simulink model "watertank_inport_NN_cex"  (R2019a)
settings: Solver=FixedStepAuto  StartTime=0.0  StopTime=options.T_train  FixedStep=0.01  RelTol=1e-3
model workspace (MAT data in the model file):
  A = 20
  a = 2
  b = 5
undefined symbols (not defined in the file): options
libraries: neural x132, simulink x5
(part 6 of 6)

== system watertank_inport_NN_cex/NN_cex_1/Layer 3/Delays 1 ==
  "p{3}" : Inport  PortDimensions=30
      mask Display: e = 0.06;c1 = [120 230 180]/255;c2 = ([120 230 180]+0)/(256+128);c3 = ([120 230 180]+128)/(256+128);patch([0 1 1 0],[0 0 1 1],c1);patch([0 1 1 1-e 1-e 0+e],[0 0 1 1-e 0+e 0+e],c2);patch([0 0 1 1-e 0+e 0+e],[0 1 1 1-e 1-e 0+e],c3);plot([0 1 1 0 0],[0 0 1 1 0]);
  mux : Mux  Inputs=1
      mask Display: e = 0.06;c1 = [120 150 230]/255;c2 = ([120 150 230]+0)/383;c3 = ([120 150 230]+128)/383;patch([0 1 1 0],[0 0 1 1],c1);patch([0 1 1 1-e 1-e 0+e],[0 0 1 1-e 0+e 0+e],c2);patch([0 0 1 1-e 0+e 0+e],[0 1 1 1-e 1-e 0+e],c3);plot([0 1 1 0 0],[0 0 1 1 0]);disp('Mux')
  "pd{3,2}" : Outport
      mask Display: e = 0.06;c1 = [120 230 180]/255;c2 = ([120 230 180]+0)/(256+128);c3 = ([120 230 180]+128)/(256+128);patch([0 1 1 0],[0 0 1 1],c1);patch([0 1 1 1-e 1-e 0+e],[0 0 1 1-e 0+e 0+e],c2);patch([0 0 1 1-e 0+e 0+e],[0 1 1 1-e 1-e 0+e],c3);plot([0 1 1 0 0],[0 0 1 1 0]);
  wires:
  "p{3}"/1 -> mux/1
  mux/1 -> "pd{3,2}"/1

== system watertank_inport_NN_cex/NN_cex_1/Layer 3/LW{3,2} ==
  "ad{3,2}" : Inport  PortDimensions=30
      mask Display: e = 0.06;c1 = [120 230 180]/255;c2 = ([120 230 180]+0)/(256+128);c3 = ([120 230 180]+128)/(256+128);patch([0 1 1 0],[0 0 1 1],c1);patch([0 1 1 1-e 1-e 0+e],[0 0 1 1-e 0+e 0+e],c2);patch([0 0 1 1-e 0+e 0+e],[0 1 1 1-e 1-e 0+e],c3);plot([0 1 1 0 0],[0 0 1 1 0]);
  "IW{3,2}(1,:)'" : Constant  Value=[0.166617845555551646885561467570369131863117218017578125;0.52084911308059655965507772634737193584442138671875;-0.310050327978324158362255502652260474860668182373046875;-0.96896711656634237908036766384611837565898895263671875;-0.467796037844698975316504174770670942962169647216796875;0.148707354038448313904297037879587151110172271728515625;-0.12519386626751460855899722446338273584842681884765625;0.70304668272030912401504565423238091170787811279296875;-0.0644584662051047863062791520860628224909305572509765625;-0.109289819706699209422851026829448528587818145751953125;-0.023767828897491537210040490890605724416673183441162109375;0.10818361570607924748710360063341795466840267181396484375;-0.6112342698872466062454122948111034929752349853515625;-0.280254882961958495801724211560213007032871246337890625;0.6513035210815980580179029857390560209751129150390625;-0.380617737563821278978792861380497924983501434326171875;-0.54080783065765813955039220672915689647197723388671875;-0.1771757921639053601214897071258747018873691558837890625;0.58377104074975261216451372092706151306629180908203125;-0.72276990720721034922036096759256906807422637939453125;0.3286623779078519103080679997219704091548919677734375;0.2250800306918193383065585067015490494668483734130859375;0.265454369326529382444590510203852318227291107177734375;0.368157490418597965753377820874447934329509735107421875;0.446124720588699730239312657431582920253276824951171875;-0.36434180520652226231703707526321522891521453857421875;0.2208616491481535659691104456214816309511661529541015625;-0.3990413717939158555481071743997745215892791748046875;-0.60167604200342506004517417750321328639984130859375;-0.284633117456618289775605035174521617591381072998046875]
      mask Display: e = 0.06;c1 = [120 150 230]/255;c2 = ([120 150 230]+0)/383;c3 = ([120 150 230]+128)/383;patch([0 1 1 0],[0 0 1 1],c1);patch([0 1 1 1-e 1-e 0+e],[0 0 1 1-e 0+e 0+e],c2);patch([0 0 1 1-e 0+e 0+e],[0 1 1 1-e 1-e 0+e],c3);plot([0 1 1 0 0],[0 0 1 1 0]);disp('weights');
  Mux : Mux  Inputs=1
      mask Display: e = 0.06;c1 = [120 150 230]/255;c2 = ([120 150 230]+0)/383;c3 = ([120 150 230]+128)/383;patch([0 1 1 0],[0 0 1 1],c1);patch([0 1 1 1-e 1-e 0+e],[0 0 1 1-e 0+e 0+e],c2);patch([0 0 1 1-e 0+e 0+e],[0 1 1 1-e 1-e 0+e],c3);plot([0 1 1 0 0],[0 0 1 1 0]);disp('Mux');
  dotprod1 : neural/Weight Functions/dotprod
      settings: SourceProductName=MATLAB Runtime - Deep Learning Toolbox  SourceProductBaseCode=Missing
  "lz{3,2}" : Outport
      mask Display: e = 0.06;c1 = [120 230 180]/255;c2 = ([120 230 180]+0)/(256+128);c3 = ([120 230 180]+128)/(256+128);patch([0 1 1 0],[0 0 1 1],c1);patch([0 1 1 1-e 1-e 0+e],[0 0 1 1-e 0+e 0+e],c2);patch([0 0 1 1-e 0+e 0+e],[0 1 1 1-e 1-e 0+e],c3);plot([0 1 1 0 0],[0 0 1 1 0]);
  wires:
  "IW{3,2}(1,:)'"/1 -> dotprod1/1
  "ad{3,2}"/1 -> dotprod1/2
  dotprod1/1 -> Mux/1
  Mux/1 -> "lz{3,2}"/1
